simulink model "test_led_enable"  (R2023b)
settings: Solver=VariableStepAuto  StartTime=0.0  StopTime=50  RelTol=1e-3
settings Model: Creator=Asus  LastModifiedBy=Asus
settings OptimizationCC: ReuseModelBlockBuffer=off

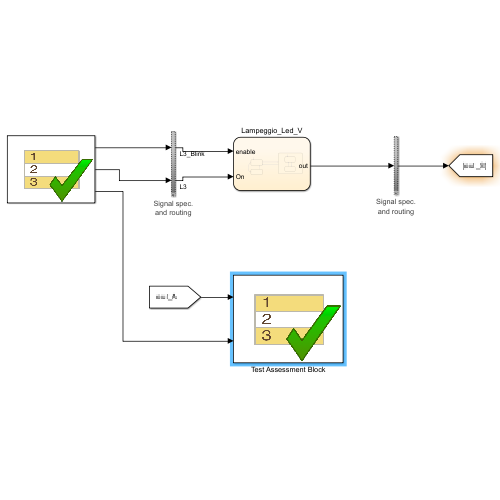
[thumbnail: Simulink's stored preview of the top-level diagram]
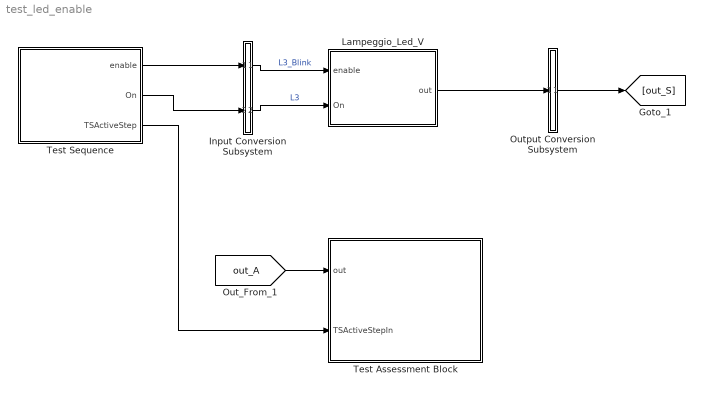
== system test_led_enable ==
  Input Conversion Subsystem : Subsystem  Tag=__SLT_ICS__  Description=|
      | Signal spec.
      | and routing
      settings: AttributesFormatString=%<Description>
  Lampeggio_Led_V : Stateflow chart  TreatAsAtomicUnit=on
  Output Conversion Subsystem : Subsystem  Tag=__SLT_OCS__  Description=|
      | Signal spec.
      | and routing
      settings: AttributesFormatString=%<Description>
  Test Assessment Block : Test Sequence  Tag=__SLT_ASMT__  TreatAsAtomicUnit=on
  Test Sequence : Test Sequence  TreatAsAtomicUnit=on
  wires:
  [out_A] -> Test Assessment Block/1(out)
  Test Sequence/1(enable) -> Input Conversion Subsystem/1(Inport_1)
  Test Sequence/2(On) -> Input Conversion Subsystem/2(Inport_2)
  Output Conversion Subsystem/1(Outport_1) -> [out_S]
  Input Conversion Subsystem/1(Outport_1) -> Lampeggio_Led_V/1(enable)  "L3_Blink"
  Input Conversion Subsystem/2(Outport_2) -> Lampeggio_Led_V/2(On)  "L3"
  Lampeggio_Led_V/1(out) -> Output Conversion Subsystem/1(Inport_1)
  Test Sequence/3(TSActiveStep) -> Test Assessment Block/2(TSActiveStepIn)

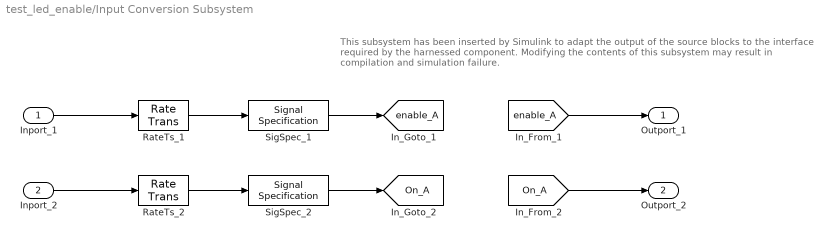
== system test_led_enable/Input Conversion Subsystem ==
  note: This subsystem has been inserted by Simulink to adapt the output of the source blocks to the interface required by the harnessed component.
      |  Modifying the contents of this subsystem may result in compilation and simulation failure.
  Inport_1 : Inport
  Inport_2 : Inport  Port=2
  RateTs_1 : RateTransition  OutPortSampleTime=[0, 1]
  RateTs_2 : RateTransition  OutPortSampleTime=[0, 1]
  SigSpec_1 : SignalSpecification  OutDataTypeStr=boolean  Dimensions=[1]  SampleTime=[0, 1]
  SigSpec_2 : SignalSpecification  OutDataTypeStr=boolean  Dimensions=[1]  SampleTime=[0, 1]
  Outport_1 : Outport
  Outport_2 : Outport  Port=2
  tag scope: On_A=global, enable_A=global
  wires:
  [enable_A] -> Outport_1/1
  SigSpec_1/1 -> [enable_A]
  RateTs_1/1 -> SigSpec_1/1
  Inport_1/1 -> RateTs_1/1
  [On_A] -> Outport_2/1
  SigSpec_2/1 -> [On_A]
  RateTs_2/1 -> SigSpec_2/1
  Inport_2/1 -> RateTs_2/1

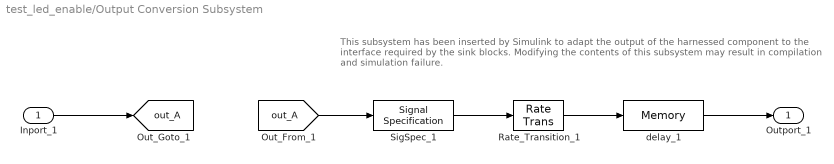
== system test_led_enable/Output Conversion Subsystem ==
  note: This subsystem has been inserted by Simulink to adapt the output of the harnessed component to the interface required by the sink blocks.
      |  Modifying the contents of this subsystem may result in compilation and simulation failure.
  Inport_1 : Inport
  Rate_Transition_1 : RateTransition  OutPortSampleTimeOpt=Inherit
  SigSpec_1 : SignalSpecification  OutDataTypeStr=boolean  Dimensions=[1]
  delay_1 : Memory
  Outport_1 : Outport
  tag scope: out_A=global
  wires:
  Inport_1/1 -> [out_A]
  [out_A] -> SigSpec_1/1
  SigSpec_1/1 -> Rate_Transition_1/1
  Rate_Transition_1/1 -> delay_1/1
  delay_1/1 -> Outport_1/1

== stateflow chart test_led_enable/Test Assessment Block ==
  state Run
    state VerifyInit
      verify(~out)
    state VerifyLedActive
      verify(out)
    state VerifyLedActive1
      verify(~out)
    state VerifyStop
      verify(~out)
    state Run_1
    (default) -> (junction 22)
    Run -> (junction 22)
    (junction 22) -> (junction 23) [order 1] : [TSActiveStepIn==TSActiveStepEnumH1.Init
        | ]
    (junction 23) -> VerifyInit [order 1] : [~in(Run.VerifyInit)]
    (junction 22) -> (junction 31) [order 2]
    (junction 23) -> (junction 26) [order 2]
    (junction 31) -> (junction 32) [order 1] : [TSActiveStepIn==TSActiveStepEnumH1.LedActive
        | ]
    (junction 32) -> VerifyLedActive [order 1] : [~in(Run.VerifyLedActive)]
    (junction 31) -> (junction 78) [order 2]
    (junction 32) -> (junction 35) [order 2]
    (junction 78) -> (junction 79) [order 1] : [TSActiveStepIn==TSActiveStepEnumH1.LedActive1
        | ]
    (junction 79) -> VerifyLedActive1 [order 1] : [~in(Run.VerifyLedActive1)]
    (junction 78) -> (junction 116) [order 2]
    (junction 79) -> (junction 82) [order 2]
    (junction 116) -> (junction 117) [order 1] : [TSActiveStepIn==TSActiveStepEnumH1.Stop
        | ]
    (junction 117) -> VerifyStop [order 1] : [~in(Run.VerifyStop)]
    (junction 116) -> (junction 60) [order 2]
    (junction 117) -> (junction 120) [order 2]
    (junction 60) -> (junction 61)
    (junction 61) -> Run_1 [order 1] : [~in(Run.Run_1)]
    (junction 61) -> (junction 64) [order 2]
  (default) -> Run
  data: out input boolean size=[1]; TSActiveStepIn input

== stateflow chart test_led_enable/Lampeggio_Led_V ==
  state blink
    state blink_on
      en: out = ACTIVE
    state blink_off
      en: out = DISACTIVE
    (default) -> blink_on
    blink_off -> blink_on : after(period, msec)
    blink_on -> blink_off : after(period, msec)
  state off
    en: out = DISACTIVE;
  state on
    en:out = ACTIVE
  (default) -> off
  off -> blink [order 1] : [enable == ACTIVE]
  off -> on [order 2] : [On==ACTIVE]
  blink -> off : [enable == DISACTIVE]
  on -> off : [On == DISACTIVE]
  data: enable input boolean; out output boolean; ACTIVE constant boolean =true; DISACTIVE constant boolean =false; period constant double =1000; On input boolean

== stateflow chart test_led_enable/Test Sequence ==
  settings: sampleTime=2.4
  state Init
    %% Initialize data outputs.
    enable = false;
    On;
    settings: description=Step iniziale il led è spento
  state LedActive
    enable=true;
    settings: description=|
        | si attiva il lampeggio del led verde per 30 secondi a una frequentìza di 1Hz
        |  (siamo nel caso in cui viene rilevata la presenza di un ostacolo a cancello chiuso o completamente aperto)
  state LedActive1
    enable=true;
    count=count+1;
    settings: description=lapeggio. contatore fino a 15 (30/2). Led un secondo acceso e uno spento
  state Stop
    enable=false;
    settings: description=Step che potrebbe essere omesso ritornanso allo Step Init
  (default) -> Init
  Init -> LedActive : [
      | true
      | ]
  LedActive -> LedActive1 : [
      | after(1,sec)
      | ]
  LedActive1 -> LedActive [order 2] : [
      | after(1,sec)
      | ]
  LedActive1 -> Stop [order 1] : [
      | count>=15
      | ]
  data: enable output boolean size=[1]; On output boolean size=[1]; TSActiveStep output Enum: TSActiveStepEnumH1; count local double [0..16] =0
